simulink model "m12sim"  (R2021b)
settings: Solver=VariableStepAuto  StartTime=0.0  StopTime=3  RelTol=1e-3
values from neighbouring files (symbols this model uses):
  K1 = wn^2    [M12.m]
  K2 = (2*zeta*wn+K1)/K1    [M12.m]
  wn = wr/sqrt(1-2*zeta^2)    [M12.m]
  zeta = rzeta(4)    [M12.m]
settings Model: Creator=Studenci  LastModifiedBy=Studenci

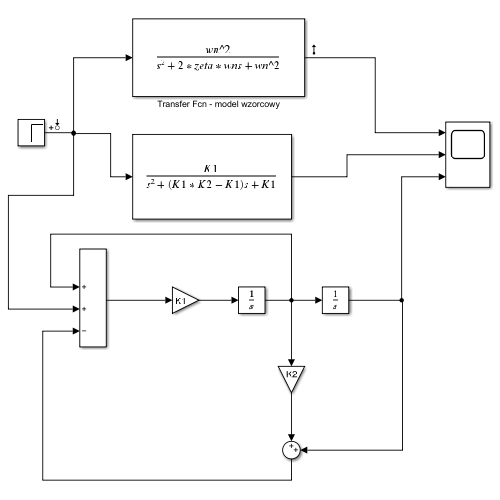
[thumbnail: Simulink's stored preview of the top-level diagram]
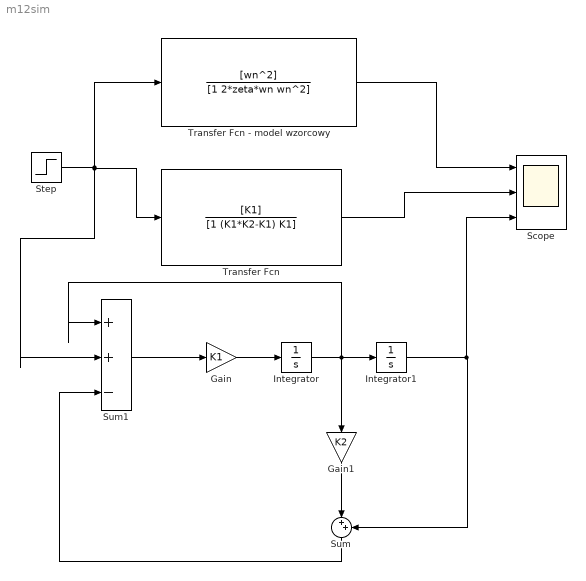
== system m12sim ==
  Gain : Gain  Gain=K1
  Gain1 : Gain  Gain=K2
  Integrator : Integrator
  Integrator1 : Integrator
  Scope : Scope  NumInputPorts=3
  Step : Step  Time=0  SampleTime=0
  Sum : Sum  Inputs=|++
  Sum1 : Sum  Inputs=|++-
  Transfer Fcn : TransferFcn  Numerator=[K1]  Denominator=[1 (K1*K2-K1) K1]
  Transfer Fcn - model wzorcowy : TransferFcn  Numerator=[wn^2]  Denominator=[1 2*zeta*wn wn^2]
  wires:
  Transfer Fcn - model wzorcowy/1 -> Scope/1
  Sum1/1 -> Gain/1
  Gain/1 -> Integrator/1
  Gain1/1 -> Sum/1
  Integrator1/1 -> Scope/3, Sum/2
  Sum/1 -> Sum1/3
  Integrator/1 -> Sum1/1, Integrator1/1, Gain1/1
  Transfer Fcn/1 -> Scope/2
  Step/1 -> Transfer Fcn/1, Sum1/2, Transfer Fcn - model wzorcowy/1
